simulink model "LBMPC_R2017b"  (R2017b)
settings: Solver=VariableStepAuto  StartTime=0.0  StopTime=6  RelTol=1e-3
values from neighbouring files (symbols this model uses):
  Ad = expm(A*dT)    [init_ctrl_design.m]    (also in init_ctrl_design_simple.m = eye(2)+A*Ts)
  Bd = (Ad-eye(n))*inv(A)*B    [init_ctrl_design.m]    (also in init_ctrl_design_simple.m = Ts*B)
  beta = 1    [TaylorRemainder.m]    (also in init_ctrl_design.m; init_ctrl_design_simple.m; mgcm_acado.m; solveMGCM.m)
  Cd = C    [init_ctrl_design.m]    (also in init_ctrl_design_simple.m = eye(2))
  Dd = D    [init_ctrl_design.m]    (also in init_ctrl_design_simple.m)
  equili = [x1; x2; x3; x4]    [TaylorRemainder.m]    (also in init_ctrl_design.m = [x1 x2 x3 x4])
  init_cond = [x1-0.35, x2-0.4, x3, 0]    [TaylorRemainder.m]    (also in init_ctrl_design.m; init_ctrl_design_simple.m = [x1-0.35, x2-0.4])
  Klqr = dlqr(Ad,Bd,Q,R)    [init_ctrl_design.m]
  Ts = 0.01    [APRBSgeneration.m]    (also in draw.m; drawCP.m = 0.1; genTrainingData.m = 0.1; init_ctrl_design.m)
  wn = sqrt(1000)    [TaylorRemainder.m]    (also in init_ctrl_design.m; mgcm_acado.m; solveMGCM.m)
  x2_c = 0    [TaylorRemainder.m]    (also in init_ctrl_design.m; init_ctrl_design_simple.m; mgcm_acado.m; solveMGCM.m)
  zeta = 1/sqrt(2)    [TaylorRemainder.m]    (also in init_ctrl_design.m; mgcm_acado.m)
undefined symbols (not defined in the file or in its folder): DiscIntNeverNeededParam, K
libraries: mpclib x1
settings Model: Creator=pbevanda  LastModifiedBy=pbevanda
settings DataIOCC: SaveFormat=Array
settings SFSimCC: SimUseLocalCustomCode=on
settings RTWCC: RTWUseLocalCustomCode=on

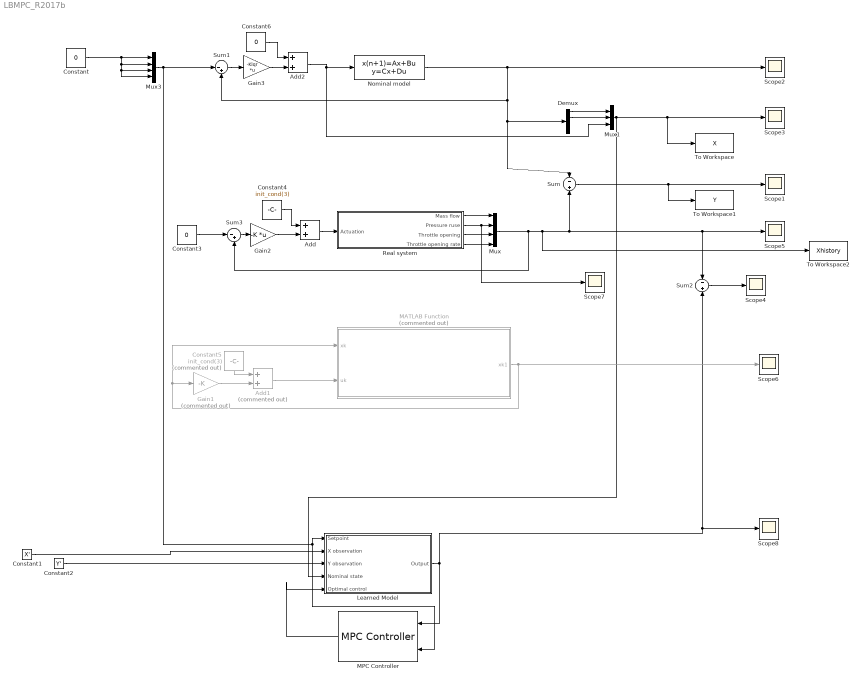
== system LBMPC_R2017b ==
  "  Nominal model" : DiscreteStateSpace  A=Ad  B=Bd  C=Cd  D=Dd  InitialCondition=equili  SampleTime=Ts
  Add : Sum
  Add1 : Sum  Commented=on
  Add2 : Sum
  Constant : Constant  Value=0
  Constant1 : Constant  Value=X'  VectorParams1D=off  SampleTime=1
  Constant2 : Constant  Value=Y'  VectorParams1D=off
  Constant3 : Constant  Value=0
  Constant4 : Constant  Value=init_cond(3)
  Constant5 : Constant  Commented=on  Value=init_cond(3)
  Constant6 : Constant  Value=0
  Demux : Demux
  Gain1 : Gain  Commented=on  Gain=-K
  Gain2 : Gain  Gain=-K  Multiplication=Matrix(K*u)
  Gain3 : Gain  Gain=-Klqr  Multiplication=Matrix(K*u)
  "Learned Model " : Subsystem
  MATLAB Function : MATLAB Function  Commented=on  TreatAsAtomicUnit=on
  MPC Controller : mpclib/MPC Controller  SCDEnableBlockLinearizationSpecification=on  is_multiple=0  enable_value=0  return_u0=off  updateMPCinCallerWorkspace=on  md_inport=off  mv_inport=off  cost_outport=off  return_sequence=off  return_qpstatus=off  return_xseq=off  return_state=off  return_ovseq=off  state_inport=off  umin_inport=off  umax_inport=off  ymin_inport=off  ymax_inport=off  cc_inport=off  ywt_inport=off  uwt_inport=off  duwt_inport=off  rhoeps_inport=off  uref_inport=off  n_ts=1  n_p=10  n_mv=1  n_md=0  n_ud=0  n_mo=4  n_uo=0  BlockDataType=double  SampleTimeInherited=off  switch_inport=off
  Mux : Mux
  Mux1 : Mux  Inputs=3
  Mux3 : Mux
  Real system : Subsystem
  Scope{1..8} (8 alike) : Scope
  Sum : Sum  Inputs=-+
  Sum1 : Sum  Inputs=|-+
  Sum2 : Sum  Inputs=-+
  Sum3 : Sum  Inputs=|-+
  To Workspace : ToWorkspace  VariableName=X  SampleTime=-1
  To Workspace1 : ToWorkspace  VariableName=Y  SampleTime=-1
  To Workspace2 : ToWorkspace  VariableName=Xhistory  SampleTime=-1
  wires:
  Demux/1 -> Mux1/1
  Real system/1("Mass flow ") -> Mux/1
  "  Nominal model"/1 -> Demux/1, Sum/1, Sum1/2, Scope2/1
  Constant/1 -> Mux3/4, Mux3/3, Mux3/2, Mux3/1
  Mux/1 -> Sum3/2, To Workspace2/1, Sum/2, Scope5/1, Sum2/1
  Sum3/1 -> Gain2/1
  Real system/4("Throttle opening rate ") -> Mux/4
  Demux/2 -> Mux1/2
  Mux3/1 -> Sum1/1, MPC Controller/2, "Learned Model "/1(Setpoint)
  Real system/2("Pressure ruse ") -> Scope7/1, Mux/2
  Add2/1 -> "  Nominal model"/1, Mux1/3
  Real system/3("Throttle opening ") -> Mux/3
  MPC Controller/1 -> "Learned Model "/5(Optimal control)
  "Learned Model "/1("Output ") -> Sum2/2, Scope8/1, MPC Controller/1
  Sum2/1 -> Scope4/1
  Sum/1 -> To Workspace1/1, Scope1/1
  Mux1/1 -> "Learned Model "/4(Nominal state), To Workspace/1, Scope3/1
  Constant2/1 -> "Learned Model "/3(Y observation)
  Constant1/1 -> "Learned Model "/2("X observation ")
  Constant3/1 -> Sum3/1
  Add/1 -> Real system/1("Actuation ")
  Gain2/1 -> Add/2
  Constant4/1 -> Add/1
  Constant5/1 -> Add1/1
  Gain1/1 -> Add1/2
  Add1/1 -> MATLAB Function/2(uk)
  MATLAB Function/1(xk1) -> Scope6/1, MATLAB Function/1(xk), Gain1/1
  Constant6/1 -> Add2/1
  Gain3/1 -> Add2/2
  Sum1/1 -> Gain3/1

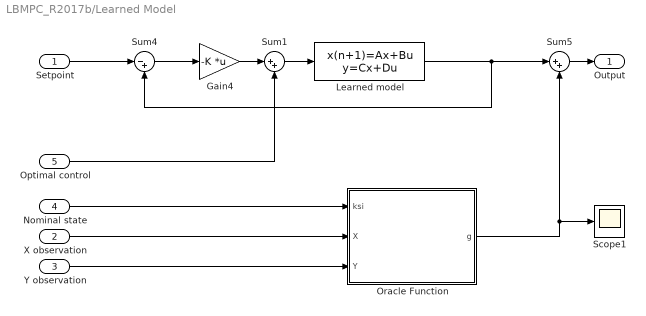
== system LBMPC_R2017b/Learned Model  ==
  Setpoint : Inport
  "X observation " : Inport  Port=2
  Y observation : Inport  Port=3
  Nominal state : Inport  Port=4
  Optimal control : Inport  Port=5
  Gain4 : Gain  Gain=-K  Multiplication=Matrix(K*u)
  Learned model : DiscreteStateSpace  A=Ad  B=Bd  C=Cd  D=Dd  InitialCondition=init_cond  SampleTime=Ts
  Oracle Function : MATLAB Function  TreatAsAtomicUnit=on
  Scope1 : Scope
  Sum1 : Sum  Inputs=|++
  Sum4 : Sum  Inputs=|-+
  Sum5 : Sum  Inputs=|++
  "Output " : Outport
  wires:
  Sum4/1 -> Gain4/1
  Learned model/1 -> Sum4/2, Sum5/1
  Setpoint/1 -> Sum4/1
  Y observation/1 -> Oracle Function/3(Y)
  "X observation "/1 -> Oracle Function/2(X)
  Nominal state/1 -> Oracle Function/1(ksi)
  Oracle Function/1(g) -> Sum5/2, Scope1/1
  Sum5/1 -> "Output "/1
  Sum1/1 -> Learned model/1
  Gain4/1 -> Sum1/1
  Optimal control/1 -> Sum1/2

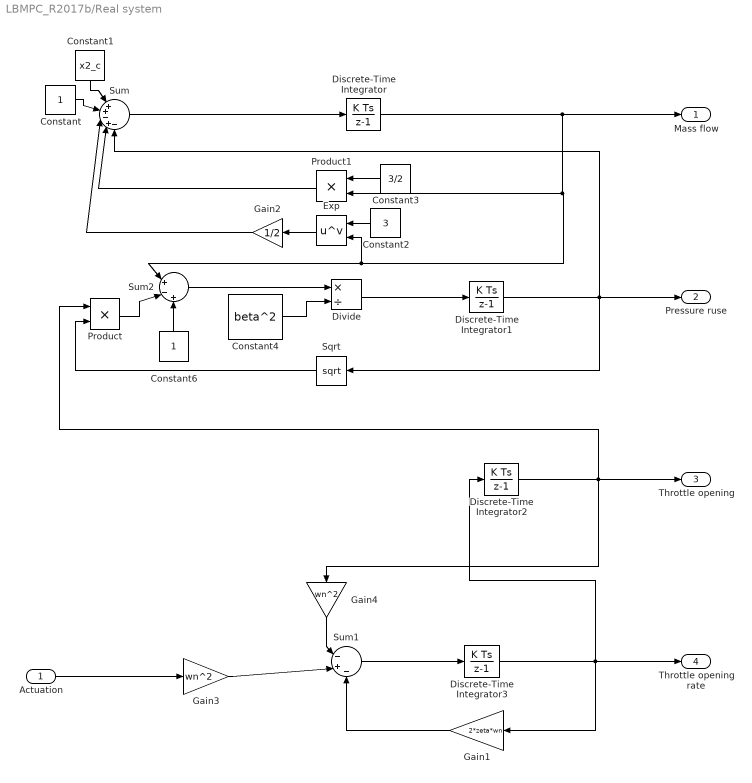
== system LBMPC_R2017b/Real system ==
  "Actuation " : Inport
  Constant : Constant
  Constant1 : Constant  Value=x2_c
  Constant2 : Constant  Value=3
  Constant3 : Constant  Value=3/2
  Constant4 : Constant  Value=beta^2
  Constant6 : Constant
  Discrete-Time Integrator : DiscreteIntegrator  InitialCondition=init_cond(1)  InitialConditionSetting=State (most efficient)  SampleTime=-1  ICPrevOutput=DiscIntNeverNeededParam  ICPrevScaledInput=DiscIntNeverNeededParam
  Discrete-Time Integrator1 : DiscreteIntegrator  InitialCondition=init_cond(2)  InitialConditionSetting=State (most efficient)  SampleTime=-1  ICPrevOutput=DiscIntNeverNeededParam  ICPrevScaledInput=DiscIntNeverNeededParam
  Discrete-Time Integrator2 : DiscreteIntegrator  InitialCondition=init_cond(3)  InitialConditionSetting=State (most efficient)  SampleTime=-1  ICPrevOutput=DiscIntNeverNeededParam  ICPrevScaledInput=DiscIntNeverNeededParam
  Discrete-Time Integrator3 : DiscreteIntegrator  InitialCondition=init_cond(4)  InitialConditionSetting=State (most efficient)  SampleTime=-1  ICPrevOutput=DiscIntNeverNeededParam  ICPrevScaledInput=DiscIntNeverNeededParam
  Divide : Product  Inputs=*/
  Exp : Math  Operator=pow  SaturateOnIntegerOverflow=on
  Gain1 : Gain  Gain=2*zeta*wn
  Gain2 : Gain  Gain=1/2
  Gain3 : Gain  Gain=wn^2
  Gain4 : Gain  Gain=wn^2
  Product : Product
  Product1 : Product
  Sqrt : Sqrt  SaturateOnIntegerOverflow=on
  Sum : Sum  Inputs=|++-+-
  Sum1 : Sum  Inputs=|-+-
  Sum2 : Sum  Inputs=|+-+
  "Mass flow " : Outport
  "Pressure ruse " : Outport  Port=2
  "Throttle opening " : Outport  Port=3
  "Throttle opening rate " : Outport  Port=4
  wires:
  Constant/1 -> Sum/2
  Constant1/1 -> Sum/1
  Constant2/1 -> Exp/1
  Constant4/1 -> Divide/2
  Sum2/1 -> Divide/1
  Constant6/1 -> Sum2/3
  Sqrt/1 -> Product/2
  Product/1 -> Sum2/2
  Divide/1 -> Discrete-Time Integrator1/1
  Exp/1 -> Gain2/1
  Gain2/1 -> Sum/3
  Constant3/1 -> Product1/1
  Product1/1 -> Sum/4
  Sum1/1 -> Discrete-Time Integrator3/1
  Gain1/1 -> Sum1/3
  Gain4/1 -> Sum1/1
  Sum/1 -> Discrete-Time Integrator/1
  Gain3/1 -> Sum1/2
  "Actuation "/1 -> Gain3/1
  Discrete-Time Integrator2/1 -> "Throttle opening "/1, Gain4/1, Product/1
  Discrete-Time Integrator3/1 -> "Throttle opening rate "/1, Discrete-Time Integrator2/1, Gain1/1
  Discrete-Time Integrator/1 -> "Mass flow "/1, Product1/2, Exp/2, Sum2/1
  Discrete-Time Integrator1/1 -> "Pressure ruse "/1, Sum/5, Sqrt/1

== matlab function LBMPC_R2017b/MATLAB Function ==
  data: xk input; xk1 output; uk input
function xk1  = trueDynamics(xk, uk)
%% Discrete-time linear dynamic model 
% 
% 4 states (x): 
%
% 1 inputs: (u)
% -------------------------------------------------------------------------
% Simulating the continuous time system
% -------------------------------------------------------------------------
% Repeat application of Euler method sampled at Ts/M.
Ts = 0.01;
M = 10;
delta = Ts/M;
xk1 = xk;
for ct=1:M
    xk1 = xk1 + delta*dynamics(xk1,uk);
end
% Note that we choose the Euler method (first oder Runge-Kutta method)
% because it is more efficient for plant with non-stiff ODEs.  You can
% choose other ODE solvers such as ode23, ode45 for better accuracy or
% ode15s and ode23s for stiff ODEs.  Those solvers are available from
% MATLAB.
end

function [f] = dynamics(x, u)
%% Continuous-time nonlinear dynamic model of a pendulum on a cart
%
% 4 states (x): 
% 
% 
% 
% 
% 
% 1 inputs: (u)
%   
%
%
% dxdt is the derivative of the states.
% [A B C D] are state space matrices linearized at the current operating point.
%
wn=sqrt(1000); % resonant frequency
zeta=1/sqrt(2); % damping coefficient
beta=1; % constant >0
x2_c=0; % pressure constant

%% Continous time state-space model of the Moore-Greitzer compressor model
f = x;
f(1) = -x(2)+x2_c+1+3*(x(1)/2)-(x(1)^3/2); % mass flow rate
f(2) = (x(1)+1-x(3)*sqrt(x(2)))/(beta^2);  % pressure rise rate
f(3) = x(4);                               % throttle opening rate
f(4) = -wn^2*x(3)-2*zeta*wn*x(4)+wn^2*u;   % throttle opening acceleration

end

== matlab function LBMPC_R2017b/Learned Model /Oracle Function ==
  data: g output; ksi input; X input; Y input
function g = oracle(ksi, X, Y)
% g = oracle(ksi, X, Y) performs a nonparametric L2 normalised Nadaraya-Watson kernel regression
if nargin <2
    X=zeros(3,1);
    Y=zeros(4,1);
end

bandwidth = 0.5;  
lambda = 0.001; 
% d = numel(ksi);
s = size(Y,1);
n = size(X,2);

kval = zeros(1,n);
for i=1:n
    % Gaussian Kernel
    kval(i) = exp(-((norm(X(:,i) - ksi).^2)/bandwidth));
end
skval = sum(kval);
weight = kval/(lambda + skval);
y=zeros(s,1);
for i=1:n
    out = weight(i)*Y(:,i);
    y = y + out;
end
g = y;
